simulink model "M5HatJoy_BLE"  (R2025b)
settings: Solver=FixedStepAuto  StartTime=0.0  StopTime=Inf  FixedStep=1/100  RelTol=1e-3  EnableMultiTasking=on
settings Model: ExtModeTrigDuration=2  Creator=totani  LastModifiedBy=totani
settings SolverCC: AutoInsertRateTranBlk=on
settings DataIOCC: SaveOutput=off  DSMLogging=off  SaveTime=off  ReturnWorkspaceOutputs=off
settings OptimizationCC: EnhancedBackFolding=on  PassReuseOutputArgsAs=Individual arguments  ZeroExternalMemoryAtStartup=off  ZeroInternalMemoryAtStartup=off  MaxStackSize=64  OptimizeBlockOrder=speed  DifferentSizesBufferReuse=on  OptimizationCustomize=off  EfficientTunableParamExpr=on
settings DebuggingCC: ParameterTunabilityLossMsg=error
settings HardwareCC: ProdBitPerPointer=32.0  ProdBitPerSizeT=32.0  ProdBitPerPtrDiffT=32.0  ProdLargestAtomicInteger=Long  ProdLargestAtomicFloat=Double  ProdWordSize=32.0  ProdHWDeviceType=ARM Compatible->ARM Cortex
settings SFSimCC: MATLABDynamicMemAlloc=off
settings RTWCC: SystemTargetFile=ert.tlc  HardwareBoard=ESP32-WROOM (Arduino Compatible)  TLCOptions="-aInlineSetEventsForThisBaseRateFcn=TLC_FALSE -aSuppressMultiTaskScheduler=TLC_FALSE  -aRateBasedStepFcn=0"  TemplateMakefile=ert_default_tmf  Toolchain=ESP32  BuildConfiguration=Faster Runs  Description=Embedded Coder
settings CodeAppCC: ForceParamTrailComments=on  IgnoreCustomStorageClasses=off  OperatorAnnotations=on  SimulinkDataObjDesc=on  SFDataObjDesc=on  InsertBlockDesc=on
settings ERTTargetCC: ExtModeTransport=3.0  ExtModeStaticAlloc=on  ExtModeAutomaticAllocSize=off  ExtModeStaticAllocSize=65536.0  ExtModeMexFile=ext_xcp  ExtModeIntrfLevel=Level2 - Open  InlinedParameterPlacement=Hierarchical  SupportContinuousTime=on  SupportVariableSizeSignals=on

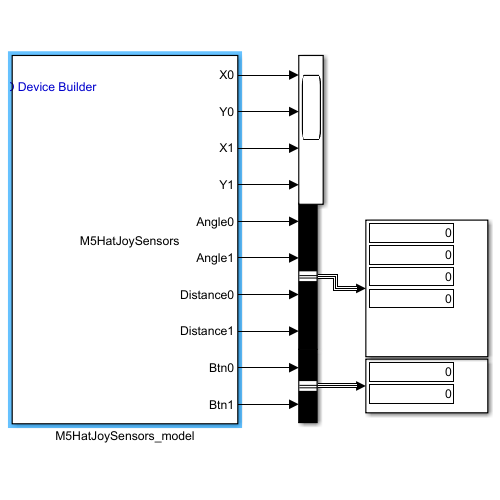
[thumbnail: Simulink's stored preview of the top-level diagram]
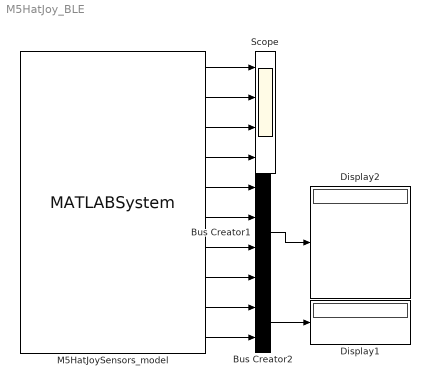
== system M5HatJoy_BLE ==
  Bus Creator1 : BusCreator  Inputs=4
  Bus Creator2 : BusCreator  Inputs=2
  Display1 : Display
  Display2 : Display
  M5HatJoySensors_model : MATLABSystem  System=M5HatJoySensors  LED_Color=0x55FF5500  SampleTime=-1
  Scope : Scope  NumInputPorts=4
      settings: ActiveDisplayYMinimum=16.750000000000004  ActiveDisplayYMaximum=199.25
  wires:
  M5HatJoySensors_model/1 -> Scope/1
  M5HatJoySensors_model/2 -> Scope/2
  M5HatJoySensors_model/3 -> Scope/3
  M5HatJoySensors_model/4 -> Scope/4
  M5HatJoySensors_model/5 -> Bus Creator1/1
  M5HatJoySensors_model/6 -> Bus Creator1/2
  M5HatJoySensors_model/7 -> Bus Creator1/3
  M5HatJoySensors_model/8 -> Bus Creator1/4
  M5HatJoySensors_model/9 -> Bus Creator2/1
  M5HatJoySensors_model/10 -> Bus Creator2/2
  Bus Creator2/1 -> Display1/1
  Bus Creator1/1 -> Display2/1
